simulink model "test"  (R2020a)
settings: Solver=FixedStepAuto  StartTime=0.0  StopTime=inf  FixedStep=.001  RelTol=1e-3  EnableMultiTasking=on
libraries: GPIO_Lib x3, USART_Lib x1, STM32_Config_Lib x1
settings Model: Creator=brunj  LastModifiedBy=tuziz
settings DataIOCC: LimitDataPoints=on  SaveFormat=Array  ReturnWorkspaceOutputs=off
settings OptimizationCC: DefaultParameterBehavior=Inlined  PassReuseOutputArgsAs=Individual arguments  LifeSpan=1  EfficientTunableParamExpr=on
settings DebuggingCC: UnderspecifiedInitializationDetection=Classic  MergeDetectMultiDrivingBlocksExec=none  SolverPrmCheckMsg=warning  AllowSymbolicDim=off  StrictBusMsg=ErrorOnBusTreatedAsVector  SFUnexpectedBacktrackingDiag=warning  SFNoUnconditionalDefaultTransitionDiag=warning  SFUndirectedBroadcastEventsDiag=error  SFExecutionAtInitializationDiag=none  ArithmeticOperatorsInVariantConditions=warning
settings HardwareCC: ProdBitPerPointer=32  ProdBitPerSizeT=32  ProdBitPerPtrDiffT=32  ProdLargestAtomicInteger=Integer  ProdWordSize=32  ProdHWDeviceType=STMicroelectronics->STM32 32-bit Cortex-M
settings ModelReferenceCC: PropagateSignalLabelsOutOfModel=off
settings SFSimCC: SimUseLocalCustomCode=off  CompileTimeRecursionLimit=0  EnableRuntimeRecursion=off  MATLABDynamicMemAlloc=off  CustomCodeUndefinedFunction=UseInterfaceOnly
settings RTWCC: Description=stm32 (Embedded Target)  SystemTargetFile=stm32.tlc  TemplateMakefile=stm32.tmf  RTWUseLocalCustomCode=off  IncludeHyperlinkInReport=on
settings CodeAppCC: IgnoreCustomStorageClasses=off  CustomSymbolStrType=$N$R$M  SimulinkBlockComments=off
settings STFCustomTargetCC: ParMdlRefBuildCompliant=on  IncludeMdlTerminateFcn=off  CombineOutputUpdateFcns=on  ERTCustomFileBanners=on  SupportNonFinite=off  SupportComplex=off  SupportContinuousTime=off  SupportNonInlinedSFcns=off  RemoveResetFunc=on  ParenthesesLevel=Maximum  CastingMode=Standards  MATLABClassNameForMDSCustomization=Simulink.SoftwareTarget.ERTCustomization  SystemTargetFile=stm32.tlc
settings ERTTargetCC: MultiwordLength=2048  CompOptLevelCompliant=off  ConcurrentExecutionCompliant=off  IncludeMdlTerminateFcn=off  SupportNonFinite=off  SupportComplex=off  ParenthesesLevel=Maximum  CastingMode=Standards  ModelStepFunctionPrototypeControlCompliant=off  CPPClassGenCompliant=off  UseToolchainInfoCompliant=off  ExtModeTransport=1  ExtModeStaticAllocSize=256  ExtModeMexArgs=0,1,115200,10  InlinedParameterPlacement=NonHierarchical  ERTSrcFileBannerTemplate=sourceFileTemplate.cgt  ERTHdrFileBannerTemplate=sourceFileTemplate.cgt  ERTDataSrcFileTemplate=sourceFileTemplate.cgt  ERTDataHdrFileTemplate=sourceFileTemplate.cgt  ERTCustomFileTemplate=customRoutineProcess.tlc  ConvertIfToSwitch=off  SuppressUnreachableDefaultCases=off  EnableSignedLeftShifts=off  EnableSignedRightShifts=off
settings ConfigComp: CovMetricSettings=dw  CovHtmlReporting=on  CovSaveCumulativeToWorkspaceVar=on  CovSaveSingleToWorkspaceVar=on  CovExternalEMLEnable=off  CovSFcnEnable=off

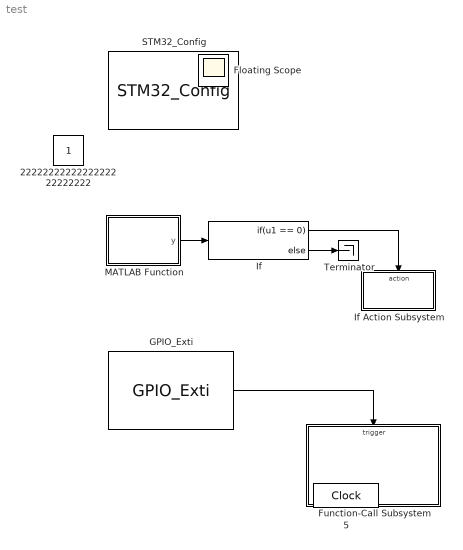
== system test ==
  Function-Call Subsystem : Subsystem  TreatAsAtomicUnit=on
  GPIO_Exti : GPIO_Lib/GPIO_Exti  Port_name=GPIOA  Pin_0=on  Pin_1=off  Pin_2=off  Pin_3=off  Pin_4=off  Pin_5=off  Pin_6=off  Pin_7=off  Pin_8=off  Pin_9=off  Pin_10=off  Pin_11=off  Pin_12=off  Pin_13=off  Pin_14=off  Pin_15=off  PinList=GPIOA0
      settings: SourceProductName=Target Support Package - STM32 Adapter
  If : If  IfExpression=u1 == 0
  If Action Subsystem : Subsystem  TreatAsAtomicUnit=on
  MATLAB Function : MATLAB Function  TreatAsAtomicUnit=on
  STM32_Config : STM32_Config_Lib/STM32_Config  Priority=0  Project_Path=.\  Config_File=test.ioc  MCU_Name=STM32F407VGTx
      settings: SourceProductName=Target Support Package - STM32 Adapter
  Terminator : Terminator
  2222222222222222222222222 : Constant  IOType=siggen
  5 : DigitalClock  IOType=siggen
  Floating Scope : Scope
  wires:
  MATLAB Function/1(y) -> If/1
  If/1 -> If Action Subsystem/Action
  If/2 -> Terminator/1
  GPIO_Exti/1 -> Function-Call Subsystem/Trigger

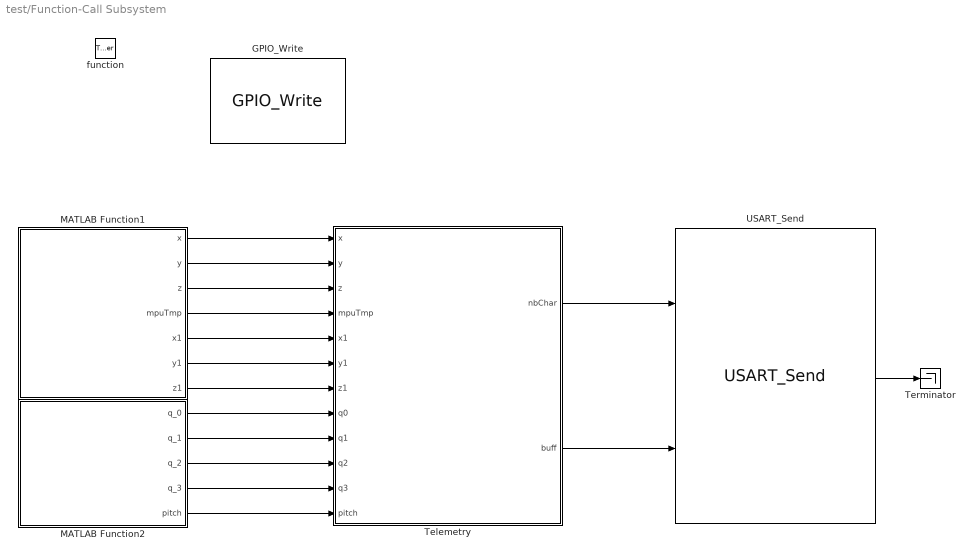
== system test/Function-Call Subsystem ==
  function : TriggerPort  TriggerType=function-call  VariantControl=Variant
  GPIO_Write : GPIO_Lib/GPIO_Write  Port_name=GPIOD  Pin0=off  Toggle_Pin0=off  Pin1=off  Toggle_Pin1=off  Pin2=off  Toggle_Pin2=off  Pin3=off  Toggle_Pin3=off  Pin4=off  Toggle_Pin4=off  Pin5=off  Toggle_Pin5=off  Pin6=off  Toggle_Pin6=off  Pin7=off  Toggle_Pin7=off  Pin8=off  Toggle_Pin8=off  Pin9=off  Toggle_Pin9=off  Pin10=off  Toggle_Pin10=off  Pin11=off  Toggle_Pin11=off  Pin12=on  Toggle_Pin12=on  Pin13=off  Toggle_Pin13=off  Pin14=off  Toggle_Pin14=off  Pin15=off  Toggle_Pin15=off  PinList="GPIOD12  13  14  15"
      settings: SourceProductName=Target Support Package - STM32 Adapter
  MATLAB Function1 : MATLAB Function  Priority=0  TreatAsAtomicUnit=on
  MATLAB Function2 : MATLAB Function  Priority=0  TreatAsAtomicUnit=on
  Telemetry : MATLAB Function  TreatAsAtomicUnit=on
  Terminator : Terminator
  USART_Send : USART_Lib/USART_Send  USART_name=USART3  Buff_size=97  nbUsart=1  usartMode=Asynchronous  usartDma_Rx=off  usartDma_Tx=off  usartIt=on
      settings: SourceProductName=Target Support Package - STM32 Adapter
  wires:
  Telemetry/2(buff) -> USART_Send/2
  Telemetry/1(nbChar) -> USART_Send/1
  USART_Send/1 -> Terminator/1
  MATLAB Function1/3(z) -> Telemetry/3(z)
  MATLAB Function1/1(x) -> Telemetry/1(x)
  MATLAB Function1/2(y) -> Telemetry/2(y)
  MATLAB Function1/4(mpuTmp) -> Telemetry/4(mpuTmp)
  MATLAB Function1/5(x1) -> Telemetry/5(x1)
  MATLAB Function1/6(y1) -> Telemetry/6(y1)
  MATLAB Function1/7(z1) -> Telemetry/7(z1)
  MATLAB Function2/1(q_0) -> Telemetry/8(q0)
  MATLAB Function2/2(q_1) -> Telemetry/9(q1)
  MATLAB Function2/3(q_2) -> Telemetry/10(q2)
  MATLAB Function2/4(q_3) -> Telemetry/11(q3)
  MATLAB Function2/5(pitch) -> Telemetry/12(pitch)

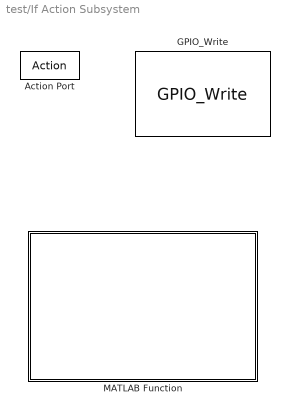
== system test/If Action Subsystem ==
  Action Port : ActionPort  ActionPortLabel=if(u1 == 0)
  GPIO_Write : GPIO_Lib/GPIO_Write  Port_name=GPIOD  Pin0=off  Toggle_Pin0=off  Pin1=off  Toggle_Pin1=off  Pin2=off  Toggle_Pin2=off  Pin3=off  Toggle_Pin3=off  Pin4=off  Toggle_Pin4=off  Pin5=off  Toggle_Pin5=off  Pin6=off  Toggle_Pin6=off  Pin7=off  Toggle_Pin7=off  Pin8=off  Toggle_Pin8=off  Pin9=off  Toggle_Pin9=off  Pin10=off  Toggle_Pin10=off  Pin11=off  Toggle_Pin11=off  Pin12=off  Toggle_Pin12=off  Pin13=on  Toggle_Pin13=on  Pin14=off  Toggle_Pin14=off  Pin15=off  Toggle_Pin15=off  PinList="GPIOD12  13  14  15"
      settings: SourceProductName=Target Support Package - STM32 Adapter
  MATLAB Function : MATLAB Function  TreatAsAtomicUnit=on

== matlab function test/Function-Call Subsystem/MATLAB Function2 ==
  data: q_0 output; q_1 output; q_2 output; q_3 output; pitch output
function [q_0,q_1,q_2,q_3,pitch]= getIMU_Values()
if coder.target('Sfun')
    % Executing in MATLAB, Buff is null
    q_0 = double(0);    
    q_1 = double(0);
    q_2 = double(0);
    q_3 = double(0);
    pitch = double(0);
else
    coder.cinclude('mpu6050.h');
    coder.cinclude('MadgwickAHRS.h');
   
    % Executing in the generated code.
    q_0 = coder.ceval('getQ_0');    
    q_1 = coder.ceval('getQ_1');
    q_2 = coder.ceval('getQ_2');
    q_3 = coder.ceval('getQ_3');
    pitch = coder.ceval('getPitch');
end

== matlab function test/MATLAB Function ==
  data: y output
function y = fcn()
if coder.target('Sfun')
    % Executing in MATLAB, Buff is null
    y = int8(0);
else
    coder.cinclude('mpu6050.h');

    % Executing in the generated code.
    y = coder.ceval('isSetup');
    
end
end

== matlab function test/Function-Call Subsystem/Telemetry ==
  data: x input; nbChar output uint16 size=1; buff output uint32 size=1; y input; z input; mpuTmp input; x1 input; y1 input; z1 input; q0 input; q1 input; q2 input; q3 input; pitch input
function [nbChar, buff] = convert(x,y,z,mpuTmp,x1,y1,z1,q0,q1,q2,q3,pitch)
if coder.target('Sfun')
    % Executing in MATLAB, Buff is null
    buff = uint32(0);
    nbChar = uint16(0);
else
    coder.cinclude('stdio.h');
    coder.cinclude('main.h');
    coder.cinclude('getBuffPtr.h');
    coder.cinclude('string.h');

    % Executing in the generated code.
    string = char(zeros(1,99));
    stringSize = uint16(size(string,2));
    stringFormat = char(['%7.3f,','%7.3f,','%7.3f,','%7.3f,','%7.3f,','%7.3f,','%7.3f,','%7.3f,','%7.3f,','%7.3f,','%7.3f,','%7.3f',13,10,0]);
    coder.ceval('snprintf',coder.wref(string),stringSize,coder.rref(stringFormat),x,y,z,mpuTmp,x1,y1,z1,q0,q1,q2,q3,pitch);
    buff = coder.ceval('getBuffPtr',coder.rref(string));
    nbChar = coder.ceval('strlen',string);
end
end

== matlab function test/If Action Subsystem/MATLAB Function ==
function fcn()
if coder.target('Sfun')
    % Executing in MATLAB, Buff is null
else
    coder.cinclude('mpu6050.h');

    % Executing in the generated code.
    coder.ceval('setFlag');
    coder.ceval('setupMPU6050');
    
end
end

== matlab function test/Function-Call Subsystem/MATLAB Function1 ==
  data: x output; y output; z output; mpuTmp output; x1 output; y1 output; z1 output
function [x,y,z,mpuTmp,x1,y1,z1]= read_mpu()
if coder.target('Sfun')
    % Executing in MATLAB, Buff is null
    x = double(0);
    y = double(0);
    z = double(0);
    mpuTmp = double(0);
    x1 = double(0);
    y1 = double(0);
    z1 = double(0);
else
    coder.cinclude('mpu6050.h');
    coder.cinclude('MadgwickAHRS.h');
    
    % Executing in the generated code.
    coder.ceval('mpu6050_read_sensors');
    
    x = coder.ceval('Accel_x_g');    
    y = coder.ceval('Accel_y_g'); 
    z = coder.ceval('Accel_z_g');
    
    mpuTmp = coder.ceval('Mpu_temp_c');
    
    x1 = coder.ceval('Gyro_x_rad');    
    y1 = coder.ceval('Gyro_y_rad'); 
    z1 = coder.ceval('Gyro_z_rad'); 
    
    coder.ceval('MadgwickAHRSupdateIMU', x1, y1, z1, x, y, z);
end
